simulink model "TRN"  (R2022a)
settings: Solver=FixedStepAuto  StartTime=0.0  StopTime=300  FixedStep=0.04  RelTol=1e-3
PreLoadFcn:
  | load('BusStructureTRNsensor.mat');
  | addpath('C:/MAP');
InitFcn:
  | %load TRNDataBusPILS.mat
  | %addpath(genpath(cd))
  | 
  | load('TPF_WHOLESIM_INPUT_SCENARIOS_AGCAS_N35_10E127_70.mat');
  | 
  | % Add DataBus Path
  | addpath(',,/');
  | addpath('../MAP/');
  | addpath('../MAP/MAP_DB');
  | addpath('../MAP/DVOF');
  | addpath(genpath(cd));
  | load('BusStructureTRN.mat');
undefined symbols (not defined in the file or in its folder): Altitude_INS, INSDataNotValid, Latitude_INS, Longitude_INS, TRN, TRNlib
libraries: simulink_extras x26, aerolibconvert2 x14, sharedtransform x3, dspstat3 x2
(part 3 of 3)

== matlab function TRN/ModeManagementCSU/TrackingCSU/GPSmode/TrackingCSU_GPS/Measurement_GPS/Fupdate_GPS ==
  data: velN input; Fmatrix output; velE input; velD input; lat input; alt input; accN input; accE input; accD input; OM input; DCMbn input; M input; N input
% ---------------------------------------------------------------------- %
%                   F matrix update function
%
%   INPUT:
%       velN: North Velocity                                [m/s]
%       velE: East Velocity                                 [m/s]
%       velD: Down Velocity                                 [m/s]
%       lat: Latitude                                       [rad]
%       alt: Altitude                                       [m]
%       accN: North acceleration                            [m/ss]
%       accE: East acceleration                             [m/ss]
%       accD: Down acceleration                             [m/ss]
%       OM: Magnitude of the rotation rate of the Earth     [rad/s]
%       R0: Radius of Earth                                 [m]
%       DCMbn: Rotational matrix(body frame to navigation frame)
%
%   OUTPUT:
%       Fmatrix: System matrix of Kalman Filter
%
% ---------------------------------------------------------------------- %
function Fmatrix = Fupdate(velN, velE, velD, lat, alt, accN, accE, accD, OM, DCMbn, M, N)
    
        Z  = zeros(3);
    
        e11 = 0;
        e12 = -((OM * sin(lat)) + (velE/(N+alt) * tan(lat)));
        e13 = velN/(M+alt);
        e21 = ((OM * sin(lat)) + (velE/(N+alt) * tan(lat)));
        e22 = 0;
        e23 = ((OM * cos(lat)) + (velE/(N+alt)));
        e31 = -velN/(M+alt);
        e32 = -(OM * cos(lat)) - (velE/(N+alt));
        e33 = 0;
        Fee = [e11 e12 e13; e21 e22 e23; e31 e32 e33;];
    
        e11 = 0;
        e12 = 1/((N+alt));
        e13 = 0;
        e21 = -1/((M+alt));
        e22 = 0 ;
        e23 = 0 ;
        e31 = 0 ;
        e32 = -tan(lat)/(N+alt) ;
        e33 = 0 ;
        Fev = [e11 e12 e13; e21 e22 e23; e31 e32 e33;];
    
        e11 = -OM * sin(lat);
        e12 = 0;
        e13 = -velE/(((N+alt))^2);
        e21 = 0 ;
        e22 = 0 ;
        e23 = velN/(((M+alt))^2);
        e31 =  -(OM*cos(lat)) - (velE/(((N+alt))*(cos(lat))^2));
        e32 = 0 ;
        e33 = (velE * tan(lat)) / ((N+alt)^2) ;
        Fep = [e11 e12 e13; e21 e22 e23; e31 e32 e33;];
    
        e11 = 0 ;
        e12 = -accD ;
        e13 = accE ;
        e21 = accD ;
        e22 = 0 ;
        e23 = -accN ;
        e31 = -accE ;
        e32 = accN ;
        e33 = 0 ;
        Fve = [e11 e12 e13; e21 e22 e23; e31 e32 e33;];
    
        e11 = velD/((M+alt));
        e12 = -2*((OM * sin(lat)) + ((velE/((N+alt))) * tan (lat))) ;
        e13 = velN/(M+alt) ;
        e21 = (2*OM * sin(lat)) + ( (velE/((N+alt))) * tan(lat) );
        e22 = (1/((N+alt))) * ((velN * tan(lat)) + velD) ;
        e23 = 2*OM * cos(lat) + (velE/((N+alt)));
        e31 = (-2*velN)/((M+alt));
        e32 = -2*(OM * cos(lat) +  (velE/((N+alt)))) ;
        e33 = 0;
        Fvv = [e11 e12 e13; e21 e22 e23; e31 e32 e33;];
    
        e11 = -velE*( (2*OM * cos(lat)) + (velE/(((N+alt))*(cos(lat))^2)));
        e12 = 0 ;
        e13 = (((velE^2)*tan(lat))/((N+alt)^2)) - ((velN*velD)/((M+alt)^2)) ;
        e21 = 2*OM *((velN*cos(lat)) - (velD*sin(lat))) + ((velN*velE) / (((N+alt))*(cos(lat))^2)) ;
        e22 = 0 ;
        e23 = ((-velE*velD)/((N+alt)^2))-((velN*velE*tan(lat))/((N+alt)^2));
        e31 = 2 * OM * velE * sin(lat);
        e32 = 0;
        e33 =  (((velE^2)/((N+alt)^2)) + ((velN^2)/((M+alt)^2)));
        Fvp = [e11 e12 e13; e21 e22 e23; e31 e32 e33;];
    
        Fpe = zeros(3);
    
        e11 = 1/((M+alt));
        e12 = 0;
        e13 = 0;
        e21 = 0;
        e22 = 1/(((N+alt))*cos(lat));
        e23 = 0;
        e31 = 0;
        e32 = 0;
        e33 = -1;
        Fpv = [e11 e12 e13; e21 e22 e23; e31 e32 e33;];
    
        e11 = 0;
        e12 = 0;
        e13 = -velN/(((M+alt))^2);
        e21 = (velE*tan(lat))/(((N+alt))*cos(lat));
        e22 = 0;
        e23 = -velE/((((N+alt))^2)*cos(lat));
        e31 = 0;
        e32 = 0;
        e33 = 0;
        Fpp = [e11 e12 e13; e21 e22 e23; e31 e32 e33;];
    
    
        %     Fvv = zeros(3);
        %     Fvp = zeros(3);
        %     Fpp = zeros(3);
    
        Fmatrix =  [Fee    Fev    Fep      DCMbn          Z      ;
                    Fve    Fvv    Fvp        Z           DCMbn   ;
                    Fpe    Fpv    Fpp        Z            Z      ;
                    Z      Z      Z          Z            Z      ;
                    Z      Z      Z          Z            Z      ;];


end

== matlab function TRN/ModeManagementCSU/TrackingCSU/GPSmode/TrackingCSU_GPS/Measurement_GPS/Gupdate_GPS ==
  data: DCMbn input; Gmatrix output
% ---------------------------------------------------------------------- %
%                   G matrix update function
%
%   INPUT:
%       DCMbn: Rotational matrix(body frame to navigation frame)
%
%   OUTPUT:
%       Gmatrix: Input matrix of Kalman Filter
%
% ---------------------------------------------------------------------- %
function Gmatrix = Gupdate(DCMbn)

Z  = zeros(3);

Gmatrix =  [ -DCMbn     Z;
                Z      DCMbn;
                Z       Z;
                Z       Z;
                Z       Z;];      

end

== matlab function TRN/ModeManagementCSU/TrackingCSU/GPSmode/TrackingCSU_GPS/Measurement_GPS/MesurementUpdate_GPS ==
  data: Lat_GPS input; Hmatrix_GPS output; Lon_GPS input; z_GPS output; alt_GPS input; velN_GPS input; velE_GPS input; velD_GPS input; Lat_INS input; Lon_INS input; alt_INS input; velN_INS input; velE_INS input; velD_INS input; M input; N input; psi input
function [Hmatrix_GPS, z_GPS] = MeasurementUpdate(Lat_GPS, Lon_GPS, alt_GPS, velN_GPS, velE_GPS, velD_GPS, ...
                                          Lat_INS, Lon_INS, alt_INS, velN_INS, velE_INS, velD_INS, ...
                                          M, N, psi)

alt = alt_INS;

Z   = zeros(3);
I   = eye(3);
H   = [(M+alt)        0             0;
         0     (N+alt)*cos(psi)     0;
         0            0             1;];

% H matrix
Hmatrix_GPS = [ Z Z H Z Z
                Z I Z Z Z]; 

z_GPS = [(M+alt)*(Lat_INS-Lat_GPS); 
    (N+alt)*cos(psi)*(Lon_INS-Lon_GPS);
     alt_INS - alt_GPS;
    velN_INS - velN_GPS;
    velE_INS - velE_GPS;
    velD_INS - velD_GPS;];


end

== matlab function TRN/ModeManagementCSU/TrackingCSU/GPSmode/TrackingCSU_GPS/Measurement_GPS/MesurementValid_GPS ==
  data: z_in input; residualValid input; roll input; pitch input; z_out output; GPStimeValid input; GPStimeValid_temp input; GPS_flag input
function z_out = MesurementValid(z_in, residualValid, roll, pitch, GPStimeValid, GPStimeValid_temp, GPS_flag)

z_out = zeros(6,1);

if (residualValid == true && abs(roll) < deg2rad(15) && abs(pitch) < deg2rad(15) && (abs(GPStimeValid - GPStimeValid_temp)) > 0.000000001)
% if (abs(roll) < deg2rad(15) && abs(pitch) < deg2rad(15) && (abs(GPStimetag - GPStimetag_temp)) > 0.000000001)
    if GPS_flag == 0
        z_out = z_in;
    elseif GPS_flag == 1
        for i = 1:6
            z_out(i)=z_in(i);
            if i > 3
                z_out(i) = 0;
            end
        end
    else
        z_out = zeros(6,1);
    end
else
    z_out = zeros(6,1);
end

== matlab function TRN/ModeManagementCSU/TrackingCSU/GPSmode/TrackingCSU_GPS/Measurement_GPS/residualValidCheck/residualCheck ==
  data: residual input; sigma_3 input; residualValid output; count output; count input
function [residualValid, count] = residualCheck(residual, sigma_3, count)

if abs(residual) >= sigma_3
    count = count + 1;
else
    count = 0;
end

if count > 7
    residualValid = boolean(false);
else
    residualValid = boolean(true);
end

== matlab function TRN/ModeManagementCSU/TrackingCSU/GPSmode/TrackingCSU_GPS/TimeTagCheck ==
  data: TimeTag_Prev input; TimeTag_Prev output; GPStimeValid input; INSTimeTag input; RALTTimeTag input
function TimeTag_Prev   = TimeTagCheck(TimeTag_Prev,GPStimeValid,INSTimeTag,RALTTimeTag)


TimeTag_Prev(4) = 0;
TimeTag_Prev(5) = 0;
TimeTag_Prev(6) = 0;

if TimeTag_Prev(1) == GPStimeValid
    TimeTag_Prev(4) = 1;
end

if TimeTag_Prev(2) == INSTimeTag
    TimeTag_Prev(5) = 1;
end

if TimeTag_Prev(3) == RALTTimeTag
    TimeTag_Prev(6) = 1;
end

TimeTag_Prev(1) = GPStimeValid;
TimeTag_Prev(2) = INSTimeTag;
TimeTag_Prev(3) = RALTTimeTag;

== matlab function TRN/ModeManagementCSU/TrackingCSU/TRNmode/TrackingCSU_TRN/EKFupdate/EKFUpdate ==
  data: z input; xu output; P output; F input; H input; G input; P input; Q input; R input; dt input; residual output; latINSErrTRN output; lonINSErrTRN output; altINSErrTRN output; hUncertainty output; vUncertainty output; xu_prev input; TimeTag input
function [xu, P, residual, latINSErrTRN, lonINSErrTRN, altINSErrTRN, ...
          hUncertainty, vUncertainty] = EKFUpdate(z, F, H, G, P, Q, R, dt, xu_prev, TimeTag)

x = zeros(15,1);
I = eye(max(size(F)));

A = I + (F*dt);
Q = (A*G * Q * G'*A') .* dt;

%-------------------------------------%
% Predicts states & covariance matrix
%-------------------------------------%
xp = A * x;
Pp = (A * P * A') + Q;

%---------------------%
% Updates Kalman gain
%---------------------%
K = (Pp * H')/(R + H * Pp * H');

%----------------%
% Updates states
%----------------%
xu = xp + K * (z - H*xp);
% residual = z - H*xp;
residual = z;

%---------------------------%
% Updates covariance matrix
%---------------------------%
P = (I - K*H) * Pp * (I - K*H)' + K*R*K';


latINSErrTRN = xu(7);
lonINSErrTRN = xu(8);
altINSErrTRN = xu(9);
hUncertainty = sqrt(abs(P(7,7) + P(8,8)));
vUncertainty = sqrt(abs(P(9,9)));

if TimeTag(6) == 1
    xu = xu_prev;
    latINSErrTRN = xu(7);
    lonINSErrTRN = xu(8);
    altINSErrTRN = xu(9);
end

end

== matlab function TRN/ModeManagementCSU/TrackingCSU/TRNmode/TrackingCSU_TRN/Earth_radius ==
  data: M output; N output; Latitude_INS input; psi output
function [M, N, psi] = Earth_radius(Latitude_INS)

    a   = 6378137;          % Earth's equatorial radius
    b   = 6356752.314245;   % Earth's polar radius
    psi = Latitude_INS;     % psi(latitude_INS)
    M   = ((a*b)^2) / ( ( (a*cos(psi))^2 + (b*sin(psi))^2 )^(3/2) );    % radius  of  curvature  in  meridian
    N   = (a^2) / ( ( (a*cos(psi))^2 + (b*sin(psi))^2 )^(1/2) );        % radius  of  curvature  in  prime  vertical

end

== matlab function TRN/ModeManagementCSU/TrackingCSU/TRNmode/TrackingCSU_TRN/INS_Update_1553falt ==
  data: latINS input; latINS output; lonINS input; altINS input; velN input; velE input; velD input; TimeTag input; lonINS output; altINS output; dt input
function [latINS, lonINS, altINS] = INS_Update_1553falt(latINS, lonINS, altINS, velN, velE, velD, TimeTag, dt)

R0 = 6378000;

if TimeTag(5) == 1
    latINS = latINS + (velN * dt) * 1/(R0+altINS);
    lonINS = lonINS + (velE * dt) * 1/(R0+altINS);
    altINS = altINS + (velD * dt) * 1/(R0+altINS);
end

== matlab function TRN/ModeManagementCSU/TrackingCSU/TRNmode/TrackingCSU_TRN/Measurement/Fupdate_TRN ==
  data: velN input; Fmatrix output; velE input; velD input; lat input; alt input; accN input; accE input; accD input; OM input; DCMbn input; M input; N input
% ---------------------------------------------------------------------- %
%                   F matrix update function
%
%   INPUT:
%       velN: North Velocity                                [m/s]
%       velE: East Velocity                                 [m/s]
%       velD: Down Velocity                                 [m/s]
%       lat: Latitude                                       [rad]
%       alt: Altitude                                       [m]
%       accN: North acceleration                            [m/ss]
%       accE: East acceleration                             [m/ss]
%       accD: Down acceleration                             [m/ss]
%       OM: Magnitude of the rotation rate of the Earth     [rad/s]
%       DCMbn: Rotational matrix(body frame to navigation frame)
%
%   OUTPUT:
%       Fmatrix: System matrix of Kalman Filter
%
% ---------------------------------------------------------------------- %
function Fmatrix = Fupdate(velN, velE, velD, lat, alt, accN, accE, accD, OM, DCMbn, M, N)
    
        Z  = zeros(3);
    
        e11 = 0;
        e12 = -((OM * sin(lat)) + (velE/(N+alt) * tan(lat)));
        e13 = velN/(M+alt);
        e21 = ((OM * sin(lat)) + (velE/(N+alt) * tan(lat)));
        e22 = 0;
        e23 = ((OM * cos(lat)) + (velE/(N+alt)));
        e31 = -velN/(M+alt);
        e32 = -(OM * cos(lat)) - (velE/(N+alt));
        e33 = 0;
        Fee = [e11 e12 e13; e21 e22 e23; e31 e32 e33;];
    
        e11 = 0;
        e12 = 1/((N+alt));
        e13 = 0;
        e21 = -1/((M+alt));
        e22 = 0 ;
        e23 = 0 ;
        e31 = 0 ;
        e32 = -tan(lat)/(N+alt) ;
        e33 = 0 ;
        Fev = [e11 e12 e13; e21 e22 e23; e31 e32 e33;];
    
        e11 = -OM * sin(lat);
        e12 = 0;
        e13 = -velE/(((N+alt))^2);
        e21 = 0 ;
        e22 = 0 ;
        e23 = velN/(((M+alt))^2);
        e31 =  -(OM*cos(lat)) - (velE/(((N+alt))*(cos(lat))^2));
        e32 = 0 ;
        e33 = (velE * tan(lat)) / ((N+alt)^2) ;
        Fep = [e11 e12 e13; e21 e22 e23; e31 e32 e33;];
    
        e11 = 0 ;
        e12 = -accD ;
        e13 = accE ;
        e21 = accD ;
        e22 = 0 ;
        e23 = -accN ;
        e31 = -accE ;
        e32 = accN ;
        e33 = 0 ;
        Fve = [e11 e12 e13; e21 e22 e23; e31 e32 e33;];
    
        e11 = velD/((M+alt));
        e12 = -2*((OM * sin(lat)) + ((velE/((N+alt))) * tan (lat))) ;
        e13 = velN/(M+alt) ;
        e21 = (2*OM * sin(lat)) + ( (velE/((N+alt))) * tan(lat) );
        e22 = (1/((N+alt))) * ((velN * tan(lat)) + velD) ;
        e23 = 2*OM * cos(lat) + (velE/((N+alt)));
        e31 = (-2*velN)/((M+alt));
        e32 = -2*(OM * cos(lat) +  (velE/((N+alt)))) ;
        e33 = 0;
        Fvv = [e11 e12 e13; e21 e22 e23; e31 e32 e33;];
    
        e11 = -velE*( (2*OM * cos(lat)) + (velE/(((N+alt))*(cos(lat))^2)));
        e12 = 0 ;
        e13 = (((velE^2)*tan(lat))/((N+alt)^2)) - ((velN*velD)/((M+alt)^2)) ;
        e21 = 2*OM *((velN*cos(lat)) - (velD*sin(lat))) + ((velN*velE) / (((N+alt))*(cos(lat))^2)) ;
        e22 = 0 ;
        e23 = ((-velE*velD)/((N+alt)^2))-((velN*velE*tan(lat))/((N+alt)^2));
        e31 = 2 * OM * velE * sin(lat);
        e32 = 0;
        e33 =  (((velE^2)/((N+alt)^2)) + ((velN^2)/((M+alt)^2)));
        Fvp = [e11 e12 e13; e21 e22 e23; e31 e32 e33;];
    
        Fpe = zeros(3);
    
        e11 = 1/((M+alt));
        e12 = 0;
        e13 = 0;
        e21 = 0;
        e22 = 1/(((N+alt))*cos(lat));
        e23 = 0;
        e31 = 0;
        e32 = 0;
        e33 = -1;
        Fpv = [e11 e12 e13; e21 e22 e23; e31 e32 e33;];
    
        e11 = 0;
        e12 = 0;
        e13 = -velN/(((M+alt))^2);
        e21 = (velE*tan(lat))/(((N+alt))*cos(lat));
        e22 = 0;
        e23 = -velE/((((N+alt))^2)*cos(lat));
        e31 = 0;
        e32 = 0;
        e33 = 0;
        Fpp = [e11 e12 e13; e21 e22 e23; e31 e32 e33;];
    
    
        %     Fvv = zeros(3);
        %     Fvp = zeros(3);
        %     Fpp = zeros(3);
    
        Fmatrix =  [Fee    Fev    Fep      DCMbn          Z      ;
                    Fve    Fvv    Fvp        Z           DCMbn   ;
                    Fpe    Fpv    Fpp        Z            Z      ;
                    Z      Z      Z          Z            Z      ;
                    Z      Z      Z          Z            Z      ;];


end

== matlab function TRN/ModeManagementCSU/TrackingCSU/TRNmode/TrackingCSU_TRN/Measurement/Gupdate_TRN ==
  data: DCMbn input; Gmatrix output
% ---------------------------------------------------------------------- %
%                   G matrix update function
%
%   INPUT:
%       DCMbn: Rotational matrix(body frame to navigation frame)
%
%   OUTPUT:
%       Gmatrix: Input matrix of Kalman Filter
%
% ---------------------------------------------------------------------- %
function Gmatrix = Gupdate(DCMbn)

Z  = zeros(3);
I  = eye(3);

Gmatrix =  [ -DCMbn     Z;
                Z      DCMbn;
                Z       Z;
                Z       Z;
                Z       Z;];      

end

== matlab function TRN/ModeManagementCSU/TrackingCSU/TRNmode/TrackingCSU_TRN/Measurement/MesurementUpdate_TRN ==
  data: Hmatrix_TRN output; lat input; lon input; alt input; RALTAltitude input; z_TRN output
% function [Hmatrix, z, hDEM] = MeasurementUpdate(resolution, lat, lon, alt, RALT)
function [Hmatrix_TRN, z_TRN] = MeasurementUpdate(lat, lon, alt, RALTAltitude)
    P_low = 0.0;
    P_high = 0.0;    
    P_left = 0.0;    
    P_right = 0.0;
    hDEM = double(0.0);         
    resultDTED = uint32(1);
    resultDVOF = int32(1);

    resolution = 3 * 0.000277777777777777;

    lat = rad2deg(lat);
    lon = rad2deg(lon);
    
    resultDVOF = coder.ceval('UpdateObstList', lat, lon);
    resultDTED = coder.ceval('UpdateMapCache', lat, lon);
    
    P_low    =   coder.ceval('GetElevation', lat - resolution, lon);
    P_high   =   coder.ceval('GetElevation', lat + resolution, lon);
    P_left   =   coder.ceval('GetElevation', lat, lon - resolution);
    P_right  =   coder.ceval('GetElevation', lat, lon + resolution);
    
    hdot_lat    =   (P_high - P_low) / resolution;
    hdot_lon    =   (P_right - P_left) / resolution;
    
    % H matrix
    Hmatrix_TRN     =  [ zeros(1,6) -hdot_lat   -hdot_lon    1  zeros(1,6) ]; 
    
    hDEM = coder.ceval('GetElevation', lat, lon);
    
    z_TRN = (alt - hDEM) - RALTAltitude;

end

== matlab function TRN/ModeManagementCSU/TrackingCSU/TRNmode/TrackingCSU_TRN/Measurement/MesurementValid_TRN ==
  data: residualValid input; roll input; pitch input; z_out output; z_in input; RALTTimeTag input; RALTTimeTag_temp input
function z_out = MesurementValid(residualValid, roll, pitch, z_in, RALTTimeTag, RALTTimeTag_temp)

z_out = 0;

if (residualValid == true && abs(roll) < deg2rad(15) && abs(pitch) < deg2rad(15) && (abs(RALTTimeTag - RALTTimeTag_temp)) > 0.000000001)
% if (RALTValid == true && abs(roll) < deg2rad(15) && abs(pitch) < deg2rad(15))
    z_out = z_in;

else
    z_out = 0;
end

== matlab function TRN/ModeManagementCSU/TrackingCSU/TRNmode/TrackingCSU_TRN/Measurement/residualValidCheck/residualCheck ==
  data: residual input; sigma_3 input; residualValid output; count output; count input
function [residualValid, count] = residualCheck(residual, sigma_3, count)

if abs(residual) >= sigma_3
    count = count + 1;
else
    count = 0;
end

if count > 7
    residualValid = boolean(false);
else
    residualValid = boolean(true);
end

== matlab function TRN/ModeManagementCSU/TrackingCSU/TRNmode/TrackingCSU_TRN/TimeTagCheck ==
  data: TimeTag_Prev input; TimeTag_Prev output; GPStimeValid input; INSTimeTag input; RALTTimeTag input
function TimeTag_Prev   = TimeTagCheck(TimeTag_Prev,GPStimeValid,INSTimeTag,RALTTimeTag)


TimeTag_Prev(4) = 0;
TimeTag_Prev(5) = 0;
TimeTag_Prev(6) = 0;

if TimeTag_Prev(1) == GPStimeValid
    TimeTag_Prev(4) = 1;
end

if TimeTag_Prev(2) == INSTimeTag
    TimeTag_Prev(5) = 1;
end

if TimeTag_Prev(3) == RALTTimeTag
    TimeTag_Prev(6) = 1;
end

TimeTag_Prev(1) = GPStimeValid;
TimeTag_Prev(2) = INSTimeTag;
TimeTag_Prev(3) = RALTTimeTag;

== matlab function TRN/DataProcess1/Subsystem3/Subsystem2/ConvertPlatformToBody1 ==
  data: vecPlatformXYZ input; vecBodyXYZ output; az_deg input
function vecBodyXYZ = ConvertPlatformToBody(vecPlatformXYZ, az_deg)
%CONVERTPLATFORMTOBODY

tformMat = diag([1, -1, -1]) * rotz( -az_deg );

vecBodyXYZ = tformMat * vecPlatformXYZ;

== matlab function TRN/TRNCorrCheck ==
  data: Acq_hold input; NavigationMode input; latINS input; TRNEstOfLatErr output; lonINS input; altINS input; TRNEstOfLonErr output; TRNEstOfaltErr output; roll input; pitch input; GPSDataNotvalid input; a input; a output
function [TRNEstOfLatErr, TRNEstOfLonErr, TRNEstOfaltErr,a] = TRNCorrCheck(Acq_hold, NavigationMode, latINS, lonINS, altINS, roll, pitch, GPSDataNotvalid, a)

persistent acq_hold_flag
if(isempty(acq_hold_flag))
    acq_hold_flag = 0;
end
acq_hold_navFlag = 0;
if GPSDataNotvalid == 1
    if Acq_hold == 1
        acq_hold_flag = 1;
    elseif Acq_hold == 0 && acq_hold_flag == 1
        acq_hold_flag = 2;
    end
    if acq_hold_flag == 1 && NavigationMode == true    % Acquisition CSU
        acq_hold_navFlag = 1;
    elseif acq_hold_flag == 2 && NavigationMode == true
        acq_hold_navFlag = 1;
    elseif NavigationMode == false
        acq_hold_flag = 0;
    end
    if abs(roll) > 15 || abs(pitch) > 15 || acq_hold_navFlag == 1
        TRNEstOfLatErr_temp = latINS;
        TRNEstOfLonErr_temp = lonINS;
        TRNEstOfaltErr_temp = altINS;
        TRNEstOfLatErr = TRNEstOfLatErr_temp;
        TRNEstOfLonErr = TRNEstOfLonErr_temp;
        TRNEstOfaltErr = TRNEstOfaltErr_temp;
        a = a+1;
    else
        TRNEstOfLatErr = latINS;
        TRNEstOfLonErr = lonINS;
        TRNEstOfaltErr = altINS;
        TRNEstOfLatErr_temp = 0;
        TRNEstOfLonErr_temp = 0;
        TRNEstOfaltErr_temp = 0;
        a = 0;
    end
    
    if a == 1
        TRNEstOfLatErr = TRNEstOfLatErr_temp;
        TRNEstOfLonErr = TRNEstOfLonErr_temp;
        TRNEstOfaltErr = TRNEstOfaltErr_temp;
    end
else
    TRNEstOfLatErr = latINS;
    TRNEstOfLonErr = lonINS;
    TRNEstOfaltErr = altINS;
    a = 0;
end

== matlab function TRN/TRNvalidCheck ==
  data: INS_Mech_flag input; TRN_valid output; Latitude_INS input
function TRN_valid = TRNvalidCheck(INS_Mech_flag, Latitude_INS)

    if( abs(Latitude_INS) > 80.0)
        Latitude_INS_flag = 0;
    else
        Latitude_INS_flag = 1;
    end

    if( (INS_Mech_flag < 1) || (Latitude_INS_flag < 1))
        TRN_valid = boolean(false);
    else
        TRN_valid = boolean(true);
    end

end

== matlab function TRN/INSValidCheck/INSValidCheck ==
  data: diff_Lat input; NotValid output; diff_Lon input; GPSDataNotValid input
function NotValid  = INSValidCheck(diff_Lat,diff_Lon, GPSDataNotValid)

utm_lat2m_deg = 110961.7060516;   
utm_lon2m_deg = 89476.51124;

if GPSDataNotValid == 1
    if (abs(diff_Lat*utm_lat2m_deg) > 15 || abs(diff_Lon*utm_lon2m_deg) > 15)  % INSvalidCheck
        NotValid = boolean(true);    % INS Notvalid
    else
        NotValid = boolean(false);   % INS valid
    end
else
    NotValid = boolean(false);      % INS valid
end

== matlab function TRN/Subsystem/FTGMapCaching ==
  data: resultDTED output; resultDVOF output; lat input; lon input; hDEM output
function [resultDTED, resultDVOF, hDEM] = FTGMapCaching(lat, lon)

resultDTED = uint32(1);
resultDVOF = int32(1);
hDEM = double(0.0);                                 %%20220419

resultDVOF = coder.ceval('UpdateObstList', lat, lon);
resultDTED = coder.ceval('UpdateMapCache', lat, lon);
hDEM = coder.ceval('GetElevation', lat, lon);       %%20220419

== matlab function TRN/Subsystem/MATLAB Function ==
  data: Resolution output; Map_Size output; bottomLat output; leftLon output
function [Resolution, Map_Size, bottomLat, leftLon] = ReturnBottomLeftLatLon

Resolution = double(0.0);
Map_Size = double(0.0);

leftLon = 0.0;
leftLon = coder.ceval('ReturnLeftLon');

bottomLat = 0.0;
bottomLat = coder.ceval('ReturnBottomLat');

end

== matlab function TRN/GPSmode_Uncertainty_init/Uncertainty_init ==
  data: P input; hUncertainty output; vUncertainty output
function [hUncertainty,vUncertainty] = Uncertainty_init(P)

hUncertainty = sqrt(abs(P(7,7) + P(8,8))) * 6378000;
vUncertainty = sqrt(abs(P(9,9)));
